simulink model "Q2p2"  (R2018b)
settings: Solver=VariableStepAuto  StartTime=0.0  StopTime=30  RelTol=1e-3
values from neighbouring files (symbols this model uses):
  A = [0           1                 0                          0 ... (first row only)    [Q2.m]
  B1 = [0 1/m1 0 1/m1+1/m2]'    [Q2.m]
  B2 = [0                 0 ... (first row only)    [Q2.m]
  C = [0 0 1 0]    [Q2.m]
settings Model: Creator=Asus  LastModifiedBy=Asus

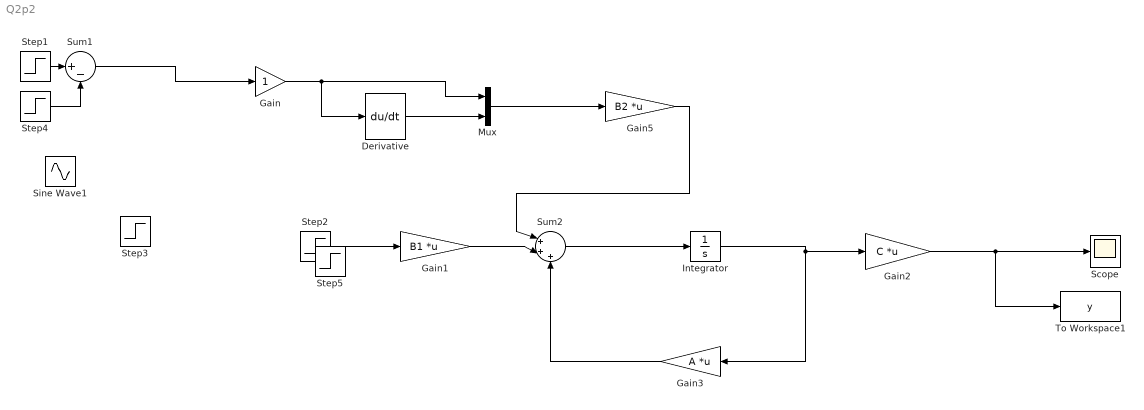
== system Q2p2 ==
  Derivative : Derivative
  Gain : Gain
  Gain1 : Gain  Gain=B1  Multiplication=Matrix(K*u) (u vector)
  Gain2 : Gain  Gain=C  Multiplication=Matrix(K*u)
  Gain3 : Gain  Gain=A  Multiplication=Matrix(K*u)
  Gain5 : Gain  Gain=B2  Multiplication=Matrix(K*u) (u vector)
  Integrator : Integrator
  Mux : Mux  Inputs=2
  Scope : Scope
  Sine Wave1 : Sin  Amplitude=0.25  Frequency=2*pi  SampleTime=0
  Step1 : Step  Time=5  After=0.25  SampleTime=0
  Step2 : Step  Time=0  After=0  SampleTime=0
  Step3 : Step  Time=0  After=0.25  SampleTime=0
  Step4 : Step  Time=10  After=0.25  SampleTime=0
  Step5 : Step  Time=0  After=0  SampleTime=0
  Sum1 : Sum  Inputs=|+-
  Sum2 : Sum  Inputs=|+++
  To Workspace1 : ToWorkspace  VariableName=y  SaveFormat=Timeseries  SampleTime=-1
  wires:
  Integrator/1 -> Gain2/1, Gain3/1
  Gain1/1 -> Sum2/2
  Gain3/1 -> Sum2/3
  Gain2/1 -> Scope/1, To Workspace1/1
  Sum2/1 -> Integrator/1
  Gain5/1 -> Sum2/1
  Step2/1 -> Gain1/1
  Mux/1 -> Gain5/1
  Step4/1 -> Sum1/2
  Derivative/1 -> Mux/2
  Gain/1 -> Derivative/1, Mux/1
  Step1/1 -> Sum1/1
  Sum1/1 -> Gain/1
